simulink model "euler_rates"  (R2017a)
settings: Solver=VariableStepAuto  StartTime=0.0  StopTime=10.0  RelTol=1e-3
settings Model: Creator=sidag  LastModifiedBy=sidag

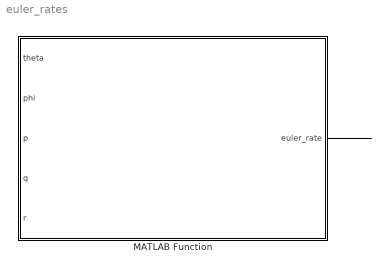
== system euler_rates ==
  MATLAB Function : MATLAB Function  TreatAsAtomicUnit=on
  wires:
  ? -> MATLAB Function/1(theta)
  ? -> MATLAB Function/2(phi)
  ? -> MATLAB Function/3(p)
  ? -> MATLAB Function/4(q)
  ? -> MATLAB Function/5(r)
  MATLAB Function/1(euler_rate) -> ?

== matlab function euler_rates/MATLAB Function ==
  data: theta input; euler_rate output; phi input; p input; q input; r input
function euler_rate = euler_rates(theta,phi,p,q,r)
%Under the following condition 
%Euler_rate=[xidot;thetadot;phidot] xidot around x thetadot around y phidot
%around z 
%Rotation is around X-Y-Z axis
%omegahatinertial=Rdot*R';
% Ris Rsb
% A comes from A*euler_rates=omegabody
%omegabody=[p;q;r]
A=[-cos(phi)*cos(theta),sin(phi),0;-cos(theta)*sin(phi),-cos(phi),0;sin(theta),0,-1];
euler_rate=(A)\[p;q;r];s
end
